simulink model "sxema"  (R2013a)
settings: Solver=ode3  StartTime=0.0  StopTime=0.6  FixedStep=0.001  RelTol=1e-3
settings Model: Creator=Huy Hung  LastModifiedBy=Huy Hung

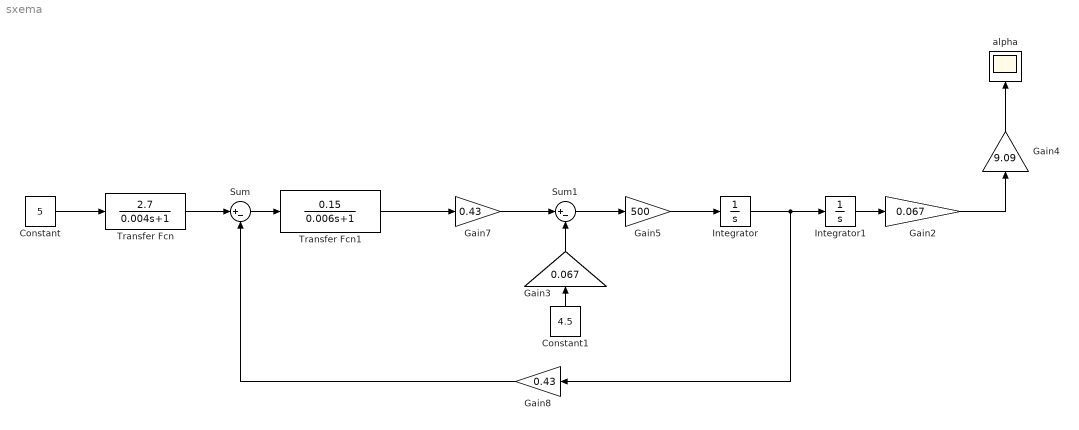
== system sxema ==
  Constant : Constant  Value=5
  Constant1 : Constant  Value=4.5
  Gain2 : Gain  Gain=0.067
  Gain3 : Gain  Gain=0.067
  Gain4 : Gain  Gain=9.09
  Gain5 : Gain  Gain=500
  Gain7 : Gain  Gain=0.43
  Gain8 : Gain  Gain=0.43
  Integrator : Integrator
  Integrator1 : Integrator
  Sum : Sum  Inputs=|+-
  Sum1 : Sum  Inputs=|+-
  Transfer Fcn : TransferFcn  Numerator=[2.7]  Denominator=[0.004 1]
  Transfer Fcn1 : TransferFcn  Numerator=[0.15]  Denominator=[0.006 1]
  alpha : Scope
      settings: SaveName=alpha
  wires:
  Constant/1 -> Transfer Fcn/1
  Transfer Fcn/1 -> Sum/1
  Sum/1 -> Transfer Fcn1/1
  Transfer Fcn1/1 -> Gain7/1
  Gain5/1 -> Integrator/1
  Integrator/1 -> Gain8/1, Integrator1/1
  Integrator1/1 -> Gain2/1
  Gain2/1 -> Gain4/1
  Gain4/1 -> alpha/1
  Gain7/1 -> Sum1/1
  Sum1/1 -> Gain5/1
  Gain3/1 -> Sum1/2
  Constant1/1 -> Gain3/1
  Gain8/1 -> Sum/2
